simulink model "desing3"  (R2024a)
settings: Solver=VariableStepAuto  StartTime=0.0  StopTime=10.0  RelTol=1e-3
libraries: spsDiodeLib x6, spsIGBTDiodeLib x6, spsThreePhaseParallelRLCBranchLib x4, spsThreePhaseVIMeasurementLib x3, spsGroundLib x2, spsSeriesRLCBranchLib x2, spsThreePhaseBreakerLib x2, spsTriangleGeneratorLib x1, spsVoltageMeasurementLib x1, spsThreePhaseProgrammableVoltageSourceLib x1, sps_lib x1
settings Model: Creator=gshma  LastModifiedBy=gshma

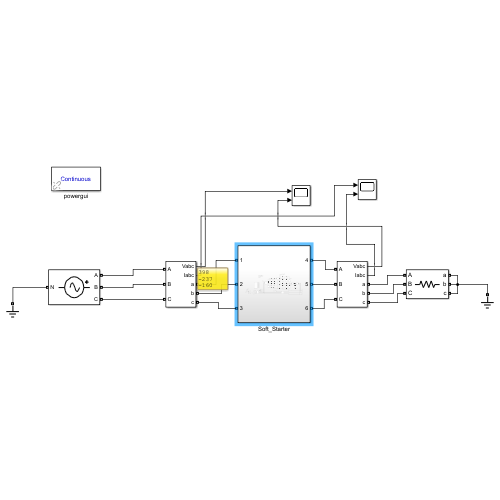
[thumbnail: Simulink's stored preview of the top-level diagram]
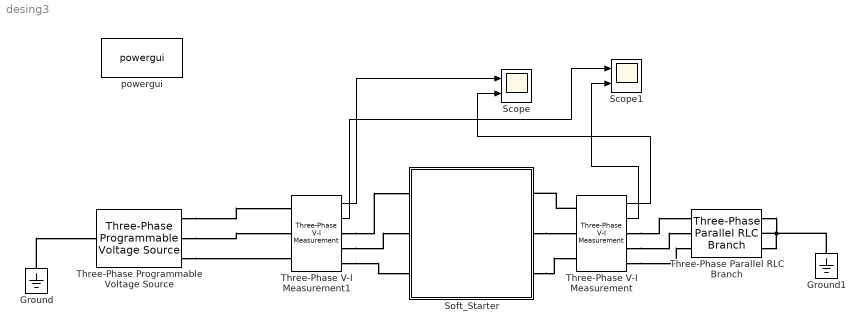
== system desing3 ==
  Ground : spsGroundLib/Ground  LConnTagsString=a
  Ground1 : spsGroundLib/Ground  LConnTagsString=a
  Scope : Scope  NumInputPorts=2
  Scope1 : Scope  NumInputPorts=2
  Soft_Starter : Subsystem
  Three-Phase Parallel RLC Branch : spsThreePhaseParallelRLCBranchLib/Three-Phase Parallel RLC Branch  LConnTagsString=A|B|C  RConnTagsString=A|B|C  BranchType=R  Resistance=10  Inductance=1e-3  Capacitance=1e-6  Measurements=None
  Three-Phase Programmable Voltage Source : spsThreePhaseProgrammableVoltageSourceLib/Three-Phase Programmable Voltage Source  PositiveSequence="[400/sqrt(2)  -30 50]"  VariationEntity=None  VariationType=Table of time-amplitude pairs  VariationTypeAlt=Step  VariationStep=0.5  VariationRate=10  VariationMagnitude=0.3  VariationFrequency=2  VariationTiming=[1 2]  VariationPhaseA=off  Amplitudes=[1 0.8 1.2 1.0]  TimeValues=[0 0.1 0.15 0.2]  HarmonicGeneration=off  HarmonicA=[3 0.2 -25 0]  HarmonicB=[2 0.15 35 2]  Timing="[0.05  3]"  BusType=swing  Pref=0  Qref=0  Qmin=-inf  Qmax=inf
  Three-Phase V-I Measurement : spsThreePhaseVIMeasurementLib/Three-Phase V-I Measurement  VoltageMeasurement=phase-to-phase  SetLabelV=off  LabelV=Vabc  Vpu=off  VpuLL=off  CurrentMeasurement=yes  SetLabelI=off  LabelI=Iabc  Ipu=off  Pbase=100e6  Vbase=500e3  OutputType=Complex  PhasorSimulation=off  PSBequivalent=0
  Three-Phase V-I Measurement1 : spsThreePhaseVIMeasurementLib/Three-Phase V-I Measurement  VoltageMeasurement=phase-to-phase  SetLabelV=off  LabelV=Vabc  Vpu=off  VpuLL=off  CurrentMeasurement=yes  SetLabelI=off  LabelI=Iabc  Ipu=off  Pbase=100e6  Vbase=500e3  OutputType=Complex  PhasorSimulation=off  PSBequivalent=0
  powergui : sps_lib/powergui  Priority=1  SimulationMode=Continuous  SampleTime=50e-6  frequency=60  Iterations=50  frequencyindice=50  Pbase=100e6  ErrMax=1e-4  UnitsV=kV  UnitsW=MW  buscounter=0  FunctionMessages=off  echomessages=off  EnableUseOfTLC=off  CurrentSourceSwitches=off  DisableSnubberDevices=off  DisableRonSwitches=off  DisableVfSwitches=off  DisplayEquations=off  AutomaticDiscreteSolvers=off  SolverType=Tustin/Backward Euler (TBE)  Interpol=off  ExternalGateDelay=off  methode=off  Ts=100  x0status=blocks  SPID=on  SwTol=0  HookPort=off  NonlinearTolerance=1e-4  nMaxIteration=100  ContinueOnMaxIteration=off  RestoreLinks=warning  ResistiveCurrentMeasurement=off  Frange=[0:2:500]  Ylog=off  Xlog=on  ShowGrid=off  save=off  variable=ZData  structure=0  ZoomFFT=off  StartTime=0.0  cycles=1  DisplayStyle=1  fundamental=60  FreqAxis=off  MaxFrequency=1000  frequencyindicesteady=1  RmsSteady=1  display=off
  wires:
  Three-Phase V-I Measurement/1 -> Scope/2
  Three-Phase V-I Measurement1/1 -> Scope/1
  Three-Phase V-I Measurement1/2 -> Scope1/1
  Three-Phase V-I Measurement/2 -> Scope1/2
  connections:
  Three-Phase Parallel RLC Branch/RConn1 -- Ground1/LConn1 -- Three-Phase Parallel RLC Branch/RConn3 -- Three-Phase Parallel RLC Branch/RConn2
  Soft_Starter/RConn2 -- Three-Phase V-I Measurement/LConn2
  Three-Phase V-I Measurement/LConn1 -- Soft_Starter/RConn1
  Three-Phase V-I Measurement/RConn1 -- Three-Phase Parallel RLC Branch/LConn1
  Three-Phase V-I Measurement/RConn2 -- Three-Phase Parallel RLC Branch/LConn2
  Three-Phase V-I Measurement/RConn3 -- Three-Phase Parallel RLC Branch/LConn3
  Three-Phase V-I Measurement1/RConn2 -- Soft_Starter/LConn2
  Three-Phase V-I Measurement1/RConn1 -- Soft_Starter/LConn1
  Three-Phase V-I Measurement1/RConn3 -- Soft_Starter/LConn3
  Soft_Starter/RConn3 -- Three-Phase V-I Measurement/LConn3
  Three-Phase Programmable Voltage Source/RConn1 -- Three-Phase V-I Measurement1/LConn1
  Three-Phase Programmable Voltage Source/RConn2 -- Three-Phase V-I Measurement1/LConn2
  Three-Phase Programmable Voltage Source/RConn3 -- Three-Phase V-I Measurement1/LConn3
  Ground/LConn1 -- Three-Phase Programmable Voltage Source/LConn1

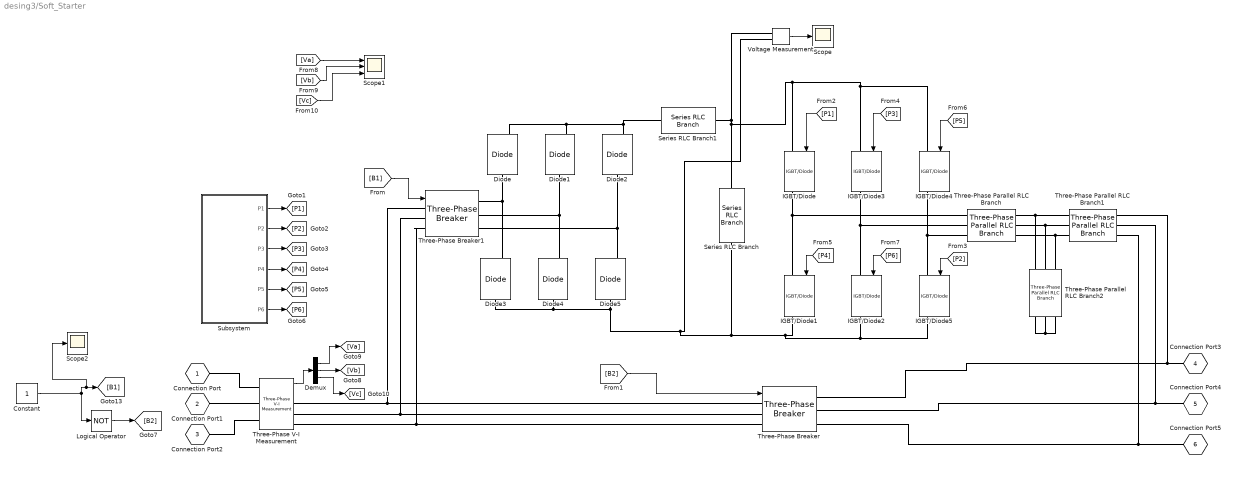
== system desing3/Soft_Starter ==
  Constant : Constant  OutDataTypeStr=boolean
  Demux : Demux  Outputs=3
  Diode{,1..5} (6 alike) : spsDiodeLib/Diode  Ron=0.001  Lon=0  Vf=0.8  IC=0  UseSnubber=0  Rs=500  Cs=250e-9  Measurements=on
  IGBT/Diode{,1..5} (6 alike) : spsIGBTDiodeLib/IGBT//Diode  Ron=1e-3  Rs=1e5  Cs=inf  Measurements=on
  Logical Operator : Logic  Operator=NOT  AllPortsSameDT=off  OutDataTypeStr=boolean
  Scope : Scope
  Scope1 : Scope  NumInputPorts=3
  Scope2 : Scope
  Series RLC Branch : spsSeriesRLCBranchLib/Series RLC Branch  LConnTagsString=__new0  RConnTagsString=__new0  BranchType=C  Resistance=1  Inductance=1e-3  SetiL0=off  InitialCurrent=0  Capacitance=7940*(10^-5)  Setx0=off  InitialVoltage=0  Measurements=None
  Series RLC Branch1 : spsSeriesRLCBranchLib/Series RLC Branch  LConnTagsString=__new0  RConnTagsString=__new0  BranchType=L  Resistance=1  Inductance=202.5*(10^-3)  SetiL0=off  InitialCurrent=0  Capacitance=4700e-6  Setx0=off  InitialVoltage=0  Measurements=None
  Subsystem : Subsystem
  Three-Phase Parallel RLC Branch : spsThreePhaseParallelRLCBranchLib/Three-Phase Parallel RLC Branch  LConnTagsString=A|B|C  RConnTagsString=A|B|C  BranchType=L  Resistance=1  Inductance=2e-3  Capacitance=1e-6  Measurements=None
  Three-Phase Parallel RLC Branch1 : spsThreePhaseParallelRLCBranchLib/Three-Phase Parallel RLC Branch  LConnTagsString=A|B|C  RConnTagsString=A|B|C  BranchType=L  Resistance=1  Inductance=4e-3  Capacitance=1e-6  Measurements=None
  Three-Phase Parallel RLC Branch2 : spsThreePhaseParallelRLCBranchLib/Three-Phase Parallel RLC Branch  LConnTagsString=A|B|C  RConnTagsString=A|B|C  BranchType=C  Resistance=2  Inductance=5e-3  Capacitance=6e-6  Measurements=None
  Three-Phase V-I Measurement : spsThreePhaseVIMeasurementLib/Three-Phase V-I Measurement  VoltageMeasurement=phase-to-phase  SetLabelV=off  LabelV=Vabc  Vpu=off  VpuLL=off  CurrentMeasurement=yes  SetLabelI=off  LabelI=Iabc  Ipu=off  Pbase=100e6  Vbase=500e3  OutputType=Complex  PhasorSimulation=off  PSBequivalent=0
  Three-Phase Breaker : spsThreePhaseBreakerLib/Three-Phase Breaker  InitialState=open  SwitchA=on  SwitchB=on  SwitchC=on  SwitchTimes="[1/60  5/60]"  External=on  BreakerResistance=0.01  SnubberResistance=1e6  SnubberCapacitance=inf  Measurements=None
  Three-Phase Breaker1 : spsThreePhaseBreakerLib/Three-Phase Breaker  InitialState=open  SwitchA=on  SwitchB=on  SwitchC=on  SwitchTimes="[1/60  5/60]"  External=on  BreakerResistance=0.01  SnubberResistance=1e6  SnubberCapacitance=inf  Measurements=None
  Voltage Measurement : spsVoltageMeasurementLib/Voltage Measurement  PhasorSimulation=off  OutputType=Complex  PSBequivalent=0
  Connection Port : PMIOPort  Tag=simrfV2util1/Connection Port  Side=Left
  Connection Port1 : PMIOPort  Tag=simrfV2util1/Connection Port  Port=2  Side=Left
  Connection Port2 : PMIOPort  Tag=simrfV2util1/Connection Port  Port=3  Side=Left
  Connection Port3 : PMIOPort  Tag=simrfV2util1/Connection Port  Port=4  Side=Right
  Connection Port4 : PMIOPort  Tag=simrfV2util1/Connection Port  Port=5  Side=Right
  Connection Port5 : PMIOPort  Tag=simrfV2util1/Connection Port  Port=6  Side=Right
  wires:
  [B2] -> Three-Phase Breaker/1
  Three-Phase V-I Measurement/1 -> Demux/1
  Demux/2 -> [Vb]
  Demux/1 -> [Va]
  Demux/3 -> [Vc]
  Constant/1 -> Scope2/1, [B1], Logical Operator/1
  Logical Operator/1 -> [B2]
  [B1] -> Three-Phase Breaker1/1
  Subsystem/2(P2) -> [P2]
  Subsystem/3(P3) -> [P3]
  Subsystem/4(P4) -> [P4]
  Subsystem/5(P5) -> [P5]
  Subsystem/6(P6) -> [P6]
  Subsystem/1(P1) -> [P1]
  [P1] -> IGBT/Diode/1
  [P2] -> IGBT/Diode5/1
  [P3] -> IGBT/Diode3/1
  [P5] -> IGBT/Diode4/1
  [P4] -> IGBT/Diode1/1
  [P6] -> IGBT/Diode2/1
  Voltage Measurement/1 -> Scope/1
  [Va] -> Scope1/1
  [Vb] -> Scope1/2
  [Vc] -> Scope1/3
  connections:
  Three-Phase V-I Measurement/RConn2 -- Three-Phase Breaker1/LConn2 -- Three-Phase Breaker/LConn2
  Three-Phase V-I Measurement/RConn1 -- Three-Phase Breaker1/LConn1 -- Three-Phase Breaker/LConn1
  Three-Phase Breaker/RConn3 -- Three-Phase Parallel RLC Branch1/RConn3 -- Connection Port5/RConn1
  Three-Phase V-I Measurement/RConn3 -- Three-Phase Breaker1/LConn3 -- Three-Phase Breaker/LConn3
  Three-Phase Breaker/RConn1 -- Three-Phase Parallel RLC Branch1/RConn1 -- Connection Port3/RConn1
  IGBT/Diode5/LConn1 -- Three-Phase Parallel RLC Branch/LConn3 -- IGBT/Diode4/RConn1
  Connection Port/RConn1 -- Three-Phase V-I Measurement/LConn1
  Connection Port1/RConn1 -- Three-Phase V-I Measurement/LConn2
  Connection Port2/RConn1 -- Three-Phase V-I Measurement/LConn3
  Diode3/RConn1 -- Diode/LConn1 -- Three-Phase Breaker1/RConn1
  Diode4/RConn1 -- Diode1/LConn1 -- Three-Phase Breaker1/RConn2
  Diode5/RConn1 -- Diode2/LConn1 -- Three-Phase Breaker1/RConn3
  IGBT/Diode/LConn1 -- Voltage Measurement/LConn1 -- Series RLC Branch1/RConn1 -- Series RLC Branch/LConn1 -- IGBT/Diode3/LConn1 -- IGBT/Diode4/LConn1
  IGBT/Diode1/RConn1 -- IGBT/Diode5/RConn1 -- IGBT/Diode2/RConn1 -- Voltage Measurement/LConn2 -- Diode4/LConn1 -- Diode3/LConn1 -- Diode5/LConn1 -- Series RLC Branch/RConn1
  Three-Phase Parallel RLC Branch/RConn2 -- Three-Phase Parallel RLC Branch2/LConn2 -- Three-Phase Parallel RLC Branch1/LConn2
  Three-Phase Parallel RLC Branch/RConn1 -- Three-Phase Parallel RLC Branch2/LConn1 -- Three-Phase Parallel RLC Branch1/LConn1
  Three-Phase Parallel RLC Branch/RConn3 -- Three-Phase Parallel RLC Branch2/LConn3 -- Three-Phase Parallel RLC Branch1/LConn3
  Three-Phase Parallel RLC Branch2/RConn1 -- Three-Phase Parallel RLC Branch2/RConn3 -- Three-Phase Parallel RLC Branch2/RConn2
  IGBT/Diode1/LConn1 -- IGBT/Diode/RConn1 -- Three-Phase Parallel RLC Branch/LConn1
  IGBT/Diode2/LConn1 -- Three-Phase Parallel RLC Branch/LConn2 -- IGBT/Diode3/RConn1
  Three-Phase Breaker/RConn2 -- Three-Phase Parallel RLC Branch1/RConn2 -- Connection Port4/RConn1
  Diode2/RConn1 -- Diode/RConn1 -- Diode1/RConn1 -- Series RLC Branch1/LConn1

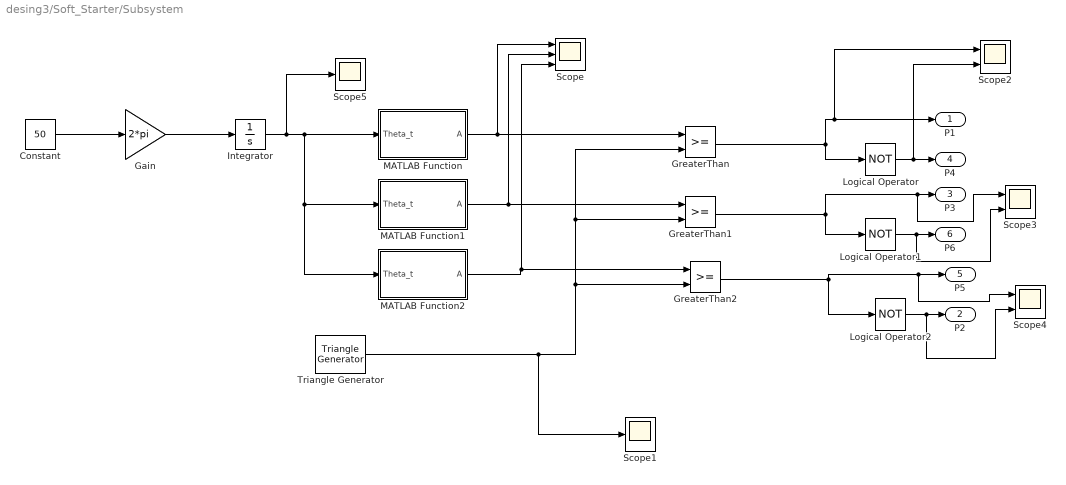
== system desing3/Soft_Starter/Subsystem ==
  Constant : Constant  Value=50
  Gain : Gain  Gain=2*pi
  GreaterThan : RelationalOperator  OutDataTypeStr=boolean  RndMeth=Simplest  InputSameDT=off
  GreaterThan1 : RelationalOperator  OutDataTypeStr=boolean  RndMeth=Simplest  InputSameDT=off
  GreaterThan2 : RelationalOperator  OutDataTypeStr=boolean  RndMeth=Simplest  InputSameDT=off
  Integrator : Integrator
  Logical Operator : Logic  Operator=NOT  AllPortsSameDT=off  OutDataTypeStr=boolean
  Logical Operator1 : Logic  Operator=NOT  AllPortsSameDT=off  OutDataTypeStr=boolean
  Logical Operator2 : Logic  Operator=NOT  AllPortsSameDT=off  OutDataTypeStr=boolean
  MATLAB Function : MATLAB Function  TreatAsAtomicUnit=on
  MATLAB Function1 : MATLAB Function  TreatAsAtomicUnit=on
  MATLAB Function2 : MATLAB Function  TreatAsAtomicUnit=on
  Scope : Scope  NumInputPorts=3
  Scope1 : Scope
  Scope2 : Scope  NumInputPorts=2
  Scope3 : Scope  NumInputPorts=2
  Scope4 : Scope  NumInputPorts=2
  Scope5 : Scope
  Triangle Generator : spsTriangleGeneratorLib/Triangle Generator  Freq=20e3  Phase=90  Ts=0
  P1 : Outport
  P2 : Outport  Port=2
  P3 : Outport  Port=3
  P4 : Outport  Port=4
  P5 : Outport  Port=5
  P6 : Outport  Port=6
  wires:
  Triangle Generator/1 -> Scope1/1, GreaterThan2/2, GreaterThan1/2, GreaterThan/2
  Constant/1 -> Gain/1
  Gain/1 -> Integrator/1
  Integrator/1 -> Scope5/1, MATLAB Function2/1(Theta_t), MATLAB Function1/1(Theta_t), MATLAB Function/1(Theta_t)
  MATLAB Function1/1(A) -> Scope/2, GreaterThan1/1
  MATLAB Function/1(A) -> Scope/1, GreaterThan/1
  MATLAB Function2/1(A) -> Scope/3, GreaterThan2/1
  GreaterThan/1 -> Scope2/1, P1/1, Logical Operator/1
  GreaterThan1/1 -> Logical Operator1/1, Scope3/1, P3/1
  GreaterThan2/1 -> Logical Operator2/1, Scope4/1, P5/1
  Logical Operator/1 -> Scope2/2, P4/1
  Logical Operator1/1 -> Scope3/2, P6/1
  Logical Operator2/1 -> Scope4/2, P2/1

== matlab function desing3/Soft_Starter/Subsystem/MATLAB Function ==
  data: Theta_t input; A output
function A = SineA(Theta_t)
A = sin(Theta_t);
end

== matlab function desing3/Soft_Starter/Subsystem/MATLAB Function2 ==
  data: Theta_t input; A output
function A = SineC(Theta_t)
A = sin(Theta_t-2*pi/3);
end

== matlab function desing3/Soft_Starter/Subsystem/MATLAB Function1 ==
  data: Theta_t input; A output
function A = SineB(Theta_t)
A = sin(Theta_t+2*pi/3);
end
